simulink model "voltage_to_fahrenheit"  (R2020b)
settings: Solver=VariableStepAuto  StartTime=0.0  StopTime=10.0  RelTol=1e-3
libraries: simulink x1
settings Model: Creator=Milind  LastModifiedBy=Milind

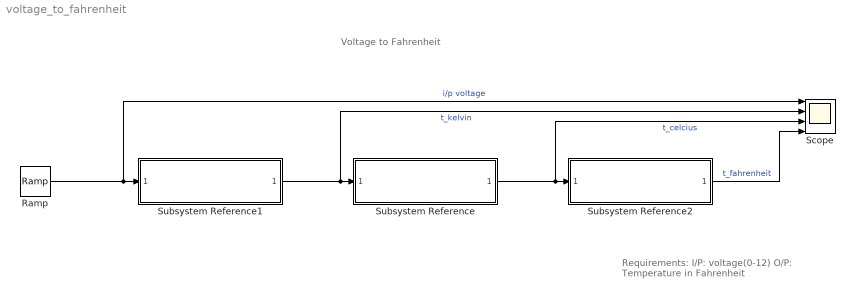
== system voltage_to_fahrenheit ==
  note: Requirements:
      | I/P: voltage(0-12)
      | O/P: Temperature in Fahrenheit
  note: Voltage to Fahrenheit
  Ramp : simulink/Sources/Ramp  slope=1  start=0  InitialOutput=0
  Scope : Scope  NumInputPorts=4
  Subsystem Reference : Subsystem  ReferencedSubsystem=kelvin_to_celcius_subsystem
  Subsystem Reference1 : Subsystem  ReferencedSubsystem=voltage_to_kelvin_subsystem
  Subsystem Reference2 : Subsystem  ReferencedSubsystem=celcius_to_fahrenheit_subsystem
  wires:
  Subsystem Reference1/1 -> Scope/2, Subsystem Reference/1  "t_kelvin"
  Subsystem Reference/1 -> Scope/3, Subsystem Reference2/1  "t_celcius"
  Ramp/1 -> Scope/1, Subsystem Reference1/1  "i/p voltage"
  Subsystem Reference2/1 -> Scope/4  "t_fahrenheit"
